simulink model "multirotor_full_system_DK"  (R2023b)
settings: Solver=VariableStepAuto  StartTime=0.0  StopTime=10.0  RelTol=1e-3
libraries: slpidlib x6
settings Model: Creator=yizho  LastModifiedBy=minu_

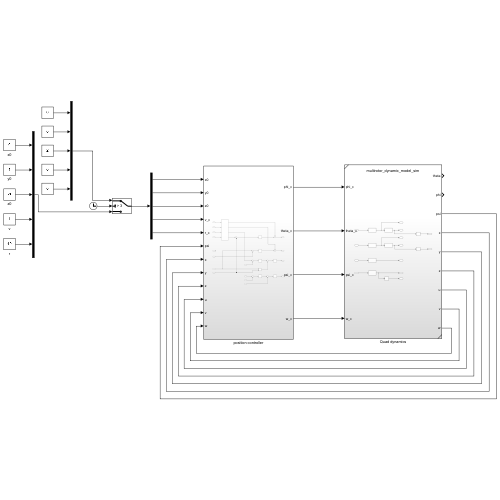
[thumbnail: Simulink's stored preview of the top-level diagram]
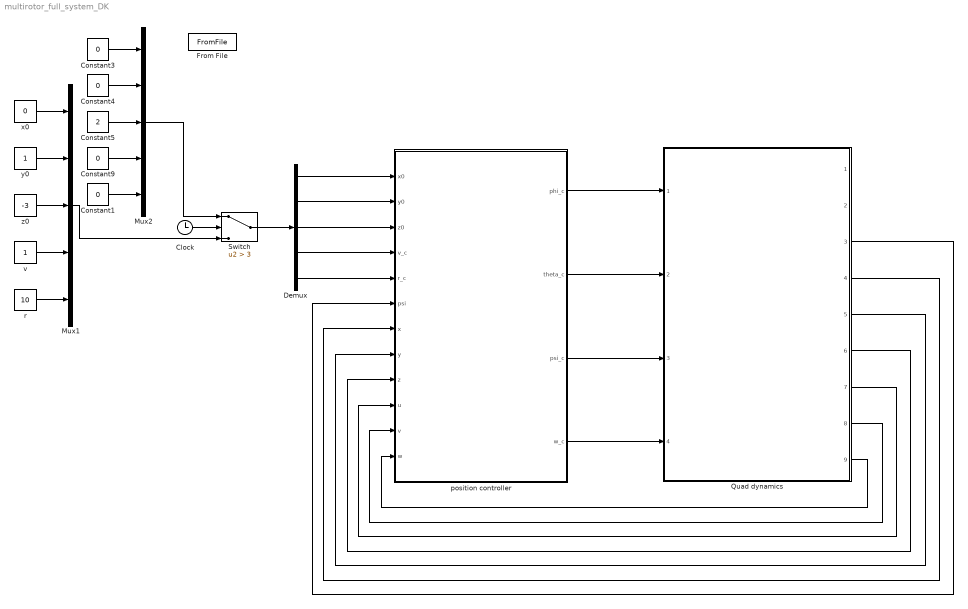
== system multirotor_full_system_DK ==
  Clock : Clock
  Constant{1,3..4,9} (4 alike) : Constant  Value=0
  Constant5 : Constant  Value=2
  Demux : Demux  Outputs=5
  Mux1 : Mux  Inputs=5
  Mux2 : Mux  Inputs=5
  Quad dynamics : Subsystem  ReferencedSubsystem=multirotor_dynamic_model_sim
  Switch : Switch  Criteria=u2 > Threshold  Threshold=3  SaturateOnIntegerOverflow=off  InputSameDT=off
  position controller : Subsystem
  r : Constant  Value=10
  v : Constant
  x0 : Constant  Value=0
  y0 : Constant
  z0 : Constant  Value=-3
  From File : FromFile  IOType=siggen  SampleTime=0
  wires:
  Clock/1 -> Switch/2
  z0/1 -> Mux1/3
  y0/1 -> Mux1/2
  x0/1 -> Mux1/1
  Switch/1 -> Demux/1
  Mux2/1 -> Switch/1
  Mux1/1 -> Switch/3
  Constant9/1 -> Mux2/4
  Constant3/1 -> Mux2/1
  Constant4/1 -> Mux2/2
  Constant5/1 -> Mux2/3
  Constant1/1 -> Mux2/5
  Demux/1 -> position controller/1(x0)
  Demux/2 -> position controller/2(y0)
  Demux/3 -> position controller/3(z0)
  position controller/1(phi_c) -> Quad dynamics/1
  position controller/2(theta_c) -> Quad dynamics/2
  position controller/3(psi_c) -> Quad dynamics/3
  position controller/4(w_c) -> Quad dynamics/4
  Quad dynamics/4 -> position controller/7(x)
  Quad dynamics/9 -> position controller/12(w)
  Quad dynamics/8 -> position controller/11(v)
  Quad dynamics/7 -> position controller/10(u)
  Quad dynamics/6 -> position controller/9(z)
  Quad dynamics/5 -> position controller/8(y)
  Quad dynamics/3 -> position controller/6(psi)
  v/1 -> Mux1/4
  r/1 -> Mux1/5
  Demux/4 -> position controller/4(v_c)
  Demux/5 -> position controller/5(r_c)

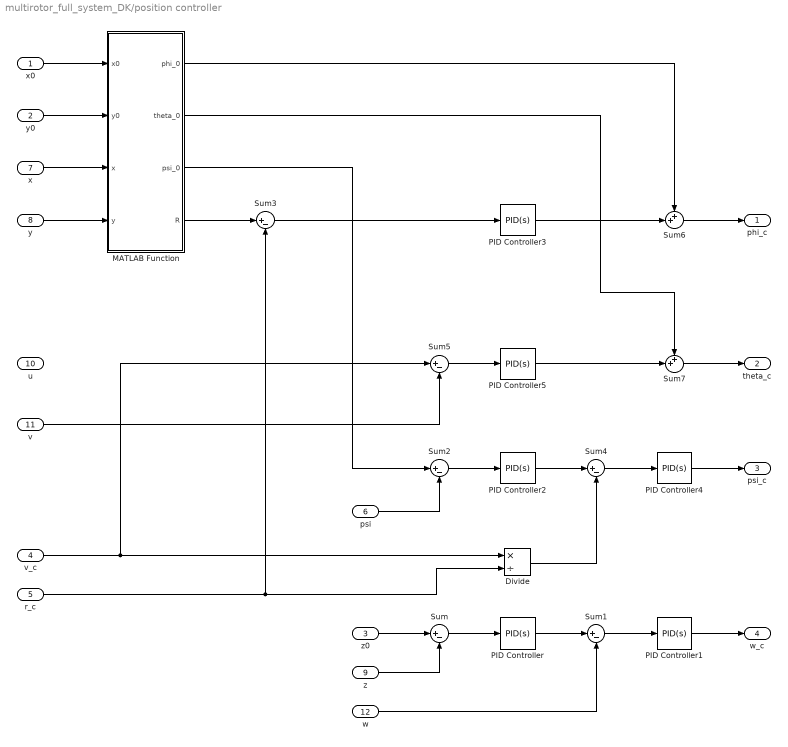
== system multirotor_full_system_DK/position controller ==
  x0 : Inport
  y0 : Inport  Port=2
  z0 : Inport  Port=3
  v_c : Inport  Port=4
  r_c : Inport  Port=5
  psi : Inport  Port=6
  x : Inport  Port=7
  y : Inport  Port=8
  z : Inport  Port=9
  u : Inport  Port=10
  v : Inport  Port=11
  w : Inport  Port=12
  Divide : Product  Inputs=*/
  MATLAB Function : MATLAB Function  TreatAsAtomicUnit=on
  PID Controller{,1..5} (6 alike) : slpidlib/PID Controller  Controller=PID  Form=Parallel  TimeDomain=Continuous-time  UseExternalTs=off  SampleTime=-1  IntegratorMethod=Forward Euler  FilterMethod=Forward Euler  ControllerParametersSource=internal  P=1  I=1  UseKiTs=off  D=0  N=100  UseFilter=on  TunerSelectOption=Transfer Function Based (PID Tuner App)  InitialConditionSource=internal  InitialConditionForIntegrator=0  InitialConditionForFilter=0  DifferentiatorICPrevScaledInput=0  ExternalReset=none  TrackingMode=off  Kt=1  LimitOutput=off  SatLimitsSource=internal  UpperSaturationLimit=inf  LowerSaturationLimit=-inf  LinearizeAsGain=on  AntiWindupMode=none  Kb=1  LimitIntegrator=off  UpperIntegratorSaturationLimit=inf  LowerIntegratorSaturationLimit=-inf  POutMin=[]  POutMax=[]  IOutMin=[]  IOutMax=[]  DOutMin=[]  DOutMax=[]  NOutMin=[]  NOutMax=[]  SumOutMin=[]  SumOutMax=[]  SaturationOutMin=[]  SaturationOutMax=[]  PParamMin=[]  PParamMax=[]  IParamMin=[]  IParamMax=[]  DParamMin=[]  DParamMax=[]  NParamMin=[]  NParamMax=[]  KbParamMin=[]  KbParamMax=[]  KtParamMin=[]  KtParamMax=[]  KbOutMin=[]  KbOutMax=[]  KtOutMin=[]  KtOutMax=[]  IntegratorOutMin=[]  IntegratorOutMax=[]  FilterOutMin=[]  FilterOutMax=[]  SumI1OutMin=[]  SumI1OutMax=[]  SumI2OutMin=[]  SumI2OutMax=[]  SumI3OutMin=[]  SumI3OutMax=[]  SumI4OutMin=[]  SumI4OutMax=[]  SumDOutMin=[]  SumDOutMax=[]  DifferentiatorOutMin=[]  DifferentiatorOutMax=[]  FilterDiffOutCoefMin=[]  FilterDiffOutCoefMax=[]  ReciprocalOutMin=[]  ReciprocalOutMax=[]  SumDenOutMin=[]  SumDenOutMax=[]  SumNumOutMin=[]  SumNumOutMax=[]  DivideOutMin=[]  DivideOutMax=[]  UdiffTsProdOutMin=[]  UdiffTsProdOutMax=[]  NTsProdOutMin=[]  NTsProdOutMax=[]  UintegralTsProdOutMin=[]  UintegralTsProdOutMax=[]  UngainTsProdOutMin=[]  UngainTsProdOutMax=[]  ClampingZeroOutDataTypeStr=Inherit: Inherit via back propagation  ClampingZeroOutMin=[]  ClampingZeroOutMax=[]  FilterDenConstantOutDataTypeStr=Inherit: Inherit via back propagation  FilterDenConstantOutMin=[]  FilterDenConstantOutMax=[]  PCopyOutDataTypeStr=Inherit: Inherit via back propagation  PCopyOutMin=[]  PCopyOutMax=[]  NCopyOutDataTypeStr=Inherit: Inherit via back propagation  NCopyOutMin=[]  NCopyOutMax=[]  IntegratorContinuousStateAttributes=''  IntegratorStateMustResolveToSignalObject=off  IntegratorRTWStateStorageClass=Auto  FilterContinuousStateAttributes=''  FilterStateMustResolveToSignalObject=off  FilterRTWStateStorageClass=Auto  ParallelPVariant=InternalParameters  IdealPVariant=Disabled  IVariant=InternalParameters  DVariant=InternalParameters  IntegratorVariant=Continuous  SatVariant=Disabled  AWVariant=Passthrough  PCopyVariant=Disabled  TRVariant=Disabled  FdbkBlocksVariant=Forward  IdealPFdbkVariant=Disabled  SatFdbkVariant=Disabled  DerivativeFilterVariant=ContFilter  NVariant=InternalParameters  NCopyVariant=Disabled  FilterICVariant=InternalICsFilter  IntegratorICVariant=InternalICs  ExternalResetVariant=Disabled  TRSumVariant=Passthrough  SumFdbkVariant=Disabled  SumVariant=Sum_PID  TsampFilterVariant=InternalTs  TsampNgainVariant=Passthrough  TsampIntegralVariant=Disabled_SignalSpec  ExternalSaturationOutDataTypeStr=Inherit: Same as second input
  Sum{,1..5} (6 alike) : Sum  Inputs=|+-
  Sum6 : Sum  Inputs=++|
  Sum7 : Sum  Inputs=++|
  phi_c : Outport
  theta_c : Outport  Port=2
  psi_c : Outport  Port=3
  w_c : Outport  Port=4
  wires:
  PID Controller/1 -> Sum1/1
  Sum/1 -> PID Controller/1
  z0/1 -> Sum/1
  z/1 -> Sum/2
  PID Controller1/1 -> w_c/1
  Sum1/1 -> PID Controller1/1
  w/1 -> Sum1/2
  psi/1 -> Sum2/2
  Sum2/1 -> PID Controller2/1
  x0/1 -> MATLAB Function/1(x0)
  y/1 -> MATLAB Function/4(y)
  x/1 -> MATLAB Function/3(x)
  y0/1 -> MATLAB Function/2(y0)
  Sum3/1 -> PID Controller3/1
  PID Controller4/1 -> psi_c/1
  v_c/1 -> Sum5/1, Divide/1
  MATLAB Function/4(R) -> Sum3/1
  Divide/1 -> Sum4/2
  PID Controller2/1 -> Sum4/1
  Sum4/1 -> PID Controller4/1
  r_c/1 -> Sum3/2, Divide/2
  PID Controller3/1 -> Sum6/2
  v/1 -> Sum5/2
  Sum5/1 -> PID Controller5/1
  PID Controller5/1 -> Sum7/2
  Sum6/1 -> phi_c/1
  Sum7/1 -> theta_c/1
  MATLAB Function/3(psi_0) -> Sum2/1
  MATLAB Function/2(theta_0) -> Sum7/1
  MATLAB Function/1(phi_0) -> Sum6/1

== matlab function multirotor_full_system_DK/position controller/MATLAB Function ==
  data: phi_0 output; theta_0 output; psi_0 output; x0 input; R output; y0 input; x input; y input
function [phi_0, theta_0, psi_0, R] = calc_angles_and_radius(x0, y0, x, y)
delta_x = x - x0;
delta_y = y - y0;
R = sqrt(delta_x^2 + delta_y^2);

% Numerical differentiation to get velocities and accelerations
dt = mean(diff(delta_x));  % Assuming constant time intervals
vx = diff(delta_x) / dt;
vy = diff(delta_y) / dt;
ax = diff(vx) / dt;
ay = diff(vy) / dt;

% Calculate curvature
curvature = (vx(1:end-1) .* ay - ax .* vy(1:end-1)) ./ (vx(1:end-1).^2 + vy(1:end-1).^2).^(3/2);

% Calculate roll angle
phi_0 = atan2(delta_y, delta_x);

% Calculate pitch angle
theta_0 = atan2(delta_y, delta_x);

% Integrate curvature to get yaw angle
psi_0 = cumtrapz(1:length(curvature), curvature);
